simulink subsystem "controller_6dof"  (R2025b)
settings: Solver=VariableStepAuto  StartTime=0.0  StopTime=10.0  RelTol=1e-3
values from neighbouring files (symbols this model uses):
  g = 9.81    [params.m]    (also in params_1dof.m; params_3dof.m)
  m = 1.210    (= 1.21)    [params.m]    (also in params_1dof.m = 1.014; params_3dof.m = 1.014)
settings Model: Creator=schwmaxi  LastModifiedBy=schwmaxi

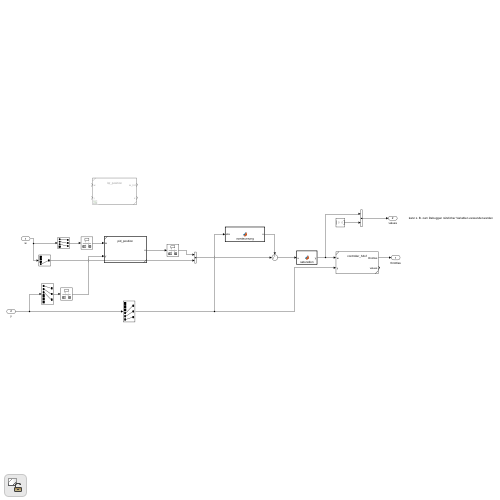
[thumbnail: Simulink's stored preview of the top-level diagram]
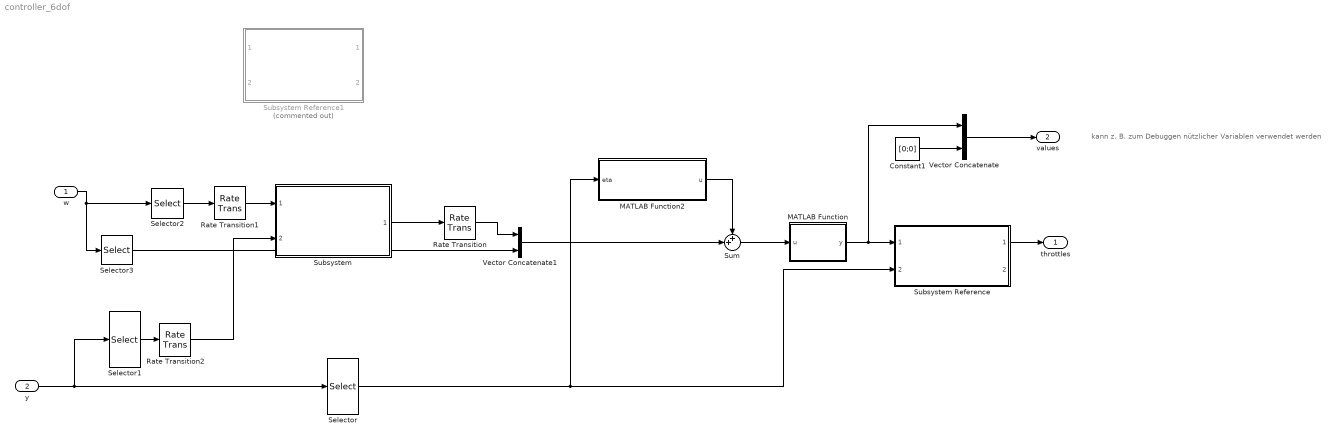
== system controller_6dof ==
  note: kann z. B. zum Debuggen nützlicher Variablen verwendet werden
  w : Inport
  y : Inport  Port=2
  Constant1 : Constant  Value=[0;0]
  MATLAB Function : MATLAB Function  TreatAsAtomicUnit=on
  MATLAB Function2 : MATLAB Function  TreatAsAtomicUnit=on
  Rate Transition : RateTransition
  Rate Transition1 : RateTransition
  Rate Transition2 : RateTransition
  Selector : Selector  InputPortWidth=6  IndexOptions=Index vector (dialog)  Indices=[4 5 6]  OutputSizes=1
  Selector1 : Selector  InputPortWidth=6  IndexOptions=Index vector (dialog)  Indices=[1 2 3]  OutputSizes=1
  Selector2 : Selector  InputPortWidth=4  IndexOptions=Index vector (dialog)  Indices=[1 2 3]  OutputSizes=1
  Selector3 : Selector  InputPortWidth=4  IndexOptions=Index vector (dialog)  Indices=[4]  OutputSizes=1
  Subsystem : Subsystem  TreatAsAtomicUnit=on  SystemSampleTime=0.02  ReferencedSubsystem=pid_position
  Subsystem Reference : Subsystem  ReferencedSubsystem=controller_3dof
  Subsystem Reference1 : Subsystem  Commented=on  TreatAsAtomicUnit=on  SystemSampleTime=0.02  ReferencedSubsystem=lqr_position
  Sum : Sum  Inputs=++|
  Vector Concatenate : Concatenate
  Vector Concatenate1 : Concatenate
  throttles : Outport
  values : Outport  Port=2
  wires:
  Selector1/1 -> Rate Transition2/1
  y/1 -> Selector/1, Selector1/1
  Selector3/1 -> Vector Concatenate1/2
  Vector Concatenate1/1 -> Sum/2
  MATLAB Function2/1(u) -> Sum/1
  Subsystem Reference/1 -> throttles/1
  Selector/1 -> MATLAB Function2/1(eta), Subsystem Reference/2
  Vector Concatenate/1 -> values/1
  Constant1/1 -> Vector Concatenate/2
  MATLAB Function/1(y) -> Vector Concatenate/1, Subsystem Reference/1
  Sum/1 -> MATLAB Function/1(u)
  Rate Transition2/1 -> Subsystem/2
  Selector2/1 -> Rate Transition1/1
  Rate Transition/1 -> Vector Concatenate1/1
  Rate Transition1/1 -> Subsystem/1
  Subsystem/1 -> Rate Transition/1
  w/1 -> Selector2/1, Selector3/1

== matlab function controller_6dof/MATLAB Function ==
  data: u input; y output
function y = saturation(u)
    y = zeros(4, 1);
    
    y(1) = min(max(u(1), -15), 15);
    y(2:3) = min(max(u(2:3), deg2rad(-5)), deg2rad(5));

== matlab function controller_6dof/MATLAB Function2 ==
  data: eta input; u output; m parameter; g parameter
function u = vorsteuerung(eta, m, g)
    u = [m * g / abs(cos(eta(1)) * cos(eta(2))); 0; 0; 0];
